simulink model "ControlObject"  (R2023a)
settings: Solver=VariableStepAuto  StartTime=0.0  StopTime=10.0  RelTol=1e-3
settings Model: Creator=romav  LastModifiedBy=romav

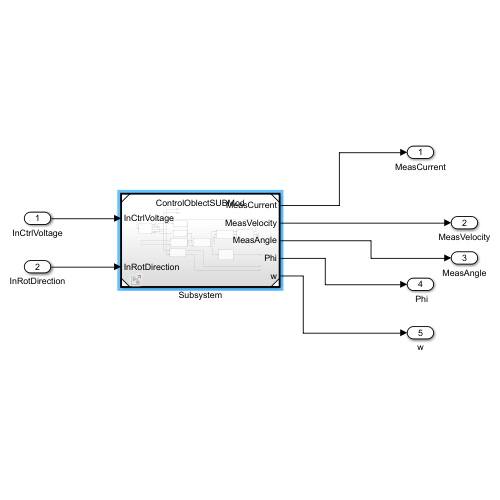
[thumbnail: Simulink's stored preview of the top-level diagram]
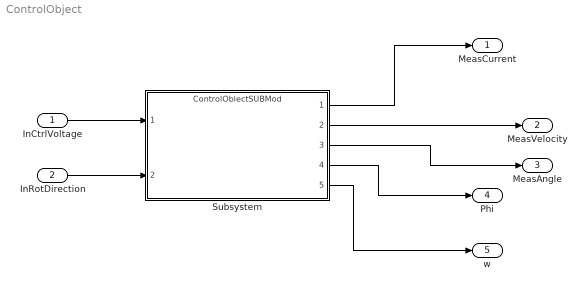
== system ControlObject ==
  InCtrlVoltage : Inport
  InRotDirection : Inport  Port=2
  Subsystem : ModelReference  ModelNameDialog=ControlOblectSUBMod  SimulationMode=Normal  ModelReferenceVersion=1.5
  MeasCurrent : Outport
  MeasVelocity : Outport  Port=2
  MeasAngle : Outport  Port=3
  " Phi" : Outport  Port=4
  w : Outport  Port=5
  wires:
  InCtrlVoltage/1 -> Subsystem/1
  InRotDirection/1 -> Subsystem/2
  Subsystem/1 -> MeasCurrent/1
  Subsystem/2 -> MeasVelocity/1
  Subsystem/3 -> MeasAngle/1
  Subsystem/4 -> " Phi"/1
  Subsystem/5 -> w/1
